simulink model "EKF_full_sim_kokany"  (R2020b)
settings: Solver=VariableStepAuto  StartTime=0.0  StopTime=1  RelTol=1e-3
settings Model: Creator=Admin  LastModifiedBy=Admin

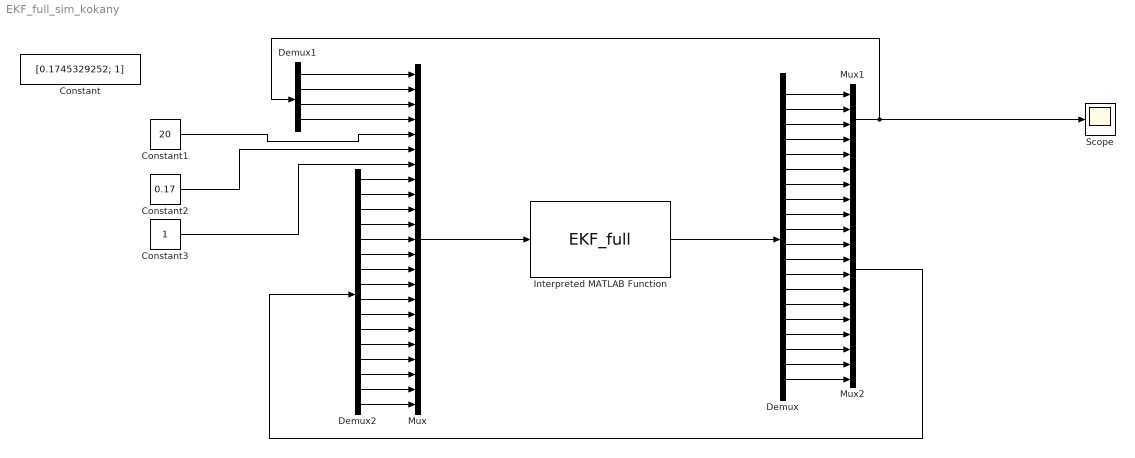
== system EKF_full_sim_kokany ==
  Constant : Constant  Value=[0.1745329252; 1]
  Constant1 : Constant  Value=20
  Constant2 : Constant  Value=0.17
  Constant3 : Constant
  Demux : Demux  Outputs=20
  Demux1 : Demux
  Demux2 : Demux  Outputs=16
  Interpreted MATLAB Function : MATLABFcn  MATLABFcn=EKF_full  OutputDimensions=20
  Mux : Mux  Inputs=23
  Mux1 : Mux
  Mux2 : Mux  Inputs=16
  Scope : Scope
  wires:
  Mux/1 -> Interpreted MATLAB Function/1
  Interpreted MATLAB Function/1 -> Demux/1
  Demux1/1 -> Mux/1
  Demux1/2 -> Mux/2
  Demux1/3 -> Mux/3
  Demux1/4 -> Mux/4
  Constant1/1 -> Mux/5
  Constant3/1 -> Mux/7
  Constant2/1 -> Mux/6
  Demux2/1 -> Mux/8
  Demux2/2 -> Mux/9
  Demux2/3 -> Mux/10
  Demux2/4 -> Mux/11
  Demux2/5 -> Mux/12
  Demux2/6 -> Mux/13
  Demux2/7 -> Mux/14
  Demux2/8 -> Mux/15
  Demux2/9 -> Mux/16
  Demux2/10 -> Mux/17
  Demux2/11 -> Mux/18
  Demux2/12 -> Mux/19
  Demux2/13 -> Mux/20
  Demux2/14 -> Mux/21
  Demux2/15 -> Mux/22
  Demux2/16 -> Mux/23
  Demux/1 -> Mux1/1
  Demux/2 -> Mux1/2
  Demux/3 -> Mux1/3
  Demux/4 -> Mux1/4
  Demux/5 -> Mux2/1
  Demux/6 -> Mux2/2
  Demux/7 -> Mux2/3
  Demux/8 -> Mux2/4
  Demux/9 -> Mux2/5
  Demux/10 -> Mux2/6
  Demux/11 -> Mux2/7
  Demux/12 -> Mux2/8
  Demux/13 -> Mux2/9
  Demux/14 -> Mux2/10
  Demux/15 -> Mux2/11
  Demux/16 -> Mux2/12
  Demux/18 -> Mux2/14
  Demux/19 -> Mux2/15
  Demux/20 -> Mux2/16
  Demux/17 -> Mux2/13
  Mux1/1 -> Demux1/1, Scope/1
  Mux2/1 -> Demux2/1
